simulink model "Script_es2"  (R2023b)
settings: Solver=VariableStepAuto  StartTime=0.0  StopTime=30  RelTol=1e-3
libraries: dspfdesign x8, vrlib x6
settings Model: PacingRate=4  Creator=bolla  LastModifiedBy=bolla

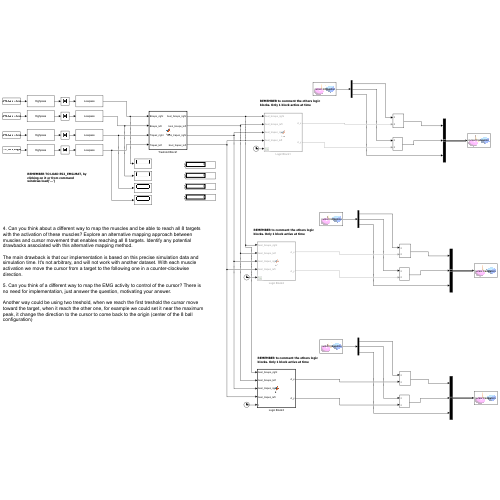
[thumbnail: Simulink's stored preview of the top-level diagram]
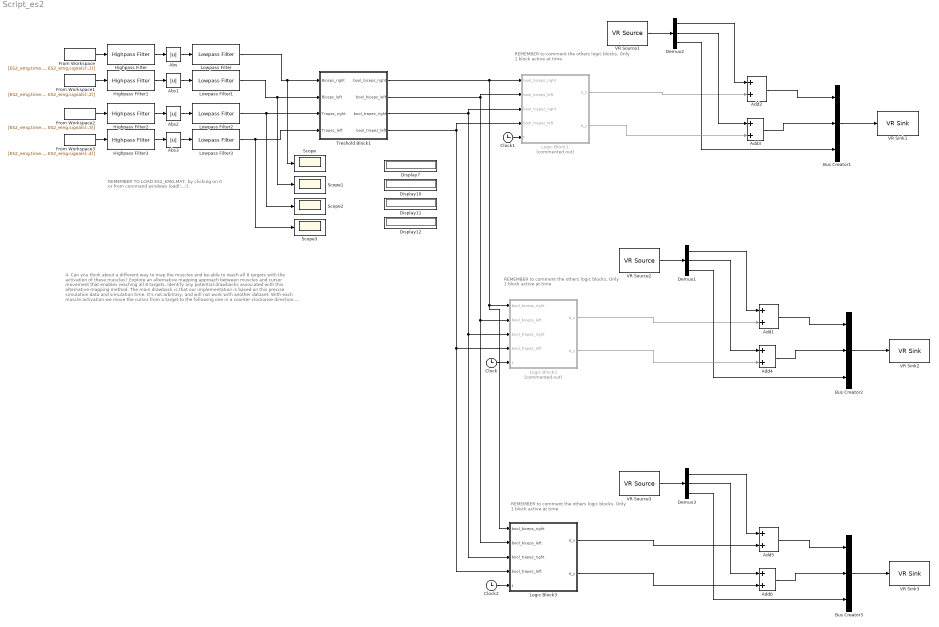
== system Script_es2 ==
  note: REMEMBER TO LOAD ES2_EMG.MAT, by clicking on it or from command windows load('...')
  note: REMEMBER to comment the others logic blocks. Only 1 block active at time
  note: 4. Can you think about a different way to map the muscles and be able to reach all 8 targets with the activation of these muscles? Explore an alternative mapping approach between muscles and cursor movement that enables reaching all 8 targets. Identify any potential drawbacks associated with this alternative mapping method.
      |
      | The main drawback is that our implementation is based on this precise simulation data and simulation time. It's not arbitrary, and will not work with another dataset. With each muscle activation we move the cursor from a target to the following one in a counter-clockwise direction.
      |
      | 5. Can you think of a different way to map the EMG activity to control of the cursor? There is no need for implementation, just answer the question, motivating your answer.
      |
      | Another way could be using two treshold, when we reach the first treshold the cursor move toward the target, when it reach the other one, for example we could set it near the maximum peak, it change the direction to the cursor to come back to the origin (center of the 8 ball configuration)
  note: REMEMBER to comment the others logic blocks. Only 1 block active at time
  note: REMEMBER to comment the others logic blocks. Only 1 block active at time
  Abs{,1..3} (4 alike) : Abs  SaturateOnIntegerOverflow=off
  Add{1..6} (6 alike) : Sum
  Bus Creator1 : BusCreator  Inputs=3
  Bus Creator2 : BusCreator  Inputs=3
  Bus Creator3 : BusCreator  Inputs=3
  Clock : Clock
  Clock1 : Clock
  Clock2 : Clock
  Demux1 : Demux  Outputs=3
  Demux2 : Demux  Outputs=3
  Demux3 : Demux  Outputs=3
  Display{7,10..12} (4 alike) : Display
  From Workspace : FromWorkspace  VariableName=[ES2_emg.time, ES2_emg.signals(:,1)]  SampleTime=0.001
  From Workspace1 : FromWorkspace  VariableName=[ES2_emg.time, ES2_emg.signals(:,2)]  SampleTime=0.001
  From Workspace2 : FromWorkspace  VariableName=[ES2_emg.time, ES2_emg.signals(:,3)]  SampleTime=0.001
  From Workspace3 : FromWorkspace  VariableName=[ES2_emg.time, ES2_emg.signals(:,4)]  SampleTime=0.001
  Highpass Filter{,1..3} (4 alike) : dspfdesign/Highpass Filter  FilterType=FIR  DesignForMinimumOrder=on  FilterOrder=50  StopbandFrequency=30  PassbandFrequency=450  StopbandAttenuation=80  PassbandRipple=0.1  SampleRate=44100  SimulateUsing=Interpreted execution  roundingMode=Floor  coeffsDataTypeStr=fixdt(1,16)
  Logic Block1 : MATLAB Function  Commented=on  TreatAsAtomicUnit=on  SystemSampleTime=0.1
  Logic Block2 : MATLAB Function  Commented=on  TreatAsAtomicUnit=on  SystemSampleTime=0.1
  Logic Block3 : MATLAB Function  TreatAsAtomicUnit=on  SystemSampleTime=0.1
  Lowpass Filter{,1..3} (4 alike) : dspfdesign/Lowpass Filter  FilterType=FIR  DesignForMinimumOrder=on  FilterOrder=50  PassbandFrequency=3  StopbandFrequency=6  PassbandRipple=0.1  StopbandAttenuation=80  SampleRate=44100  SimulateUsing=Interpreted execution  roundingMode=Floor  coeffsDataTypeStr=fixdt(1,16)
  Scope{,1..3} (4 alike) : Scope
  Treshold Block1 : MATLAB Function  TreatAsAtomicUnit=on  SystemSampleTime=0.1
  VR Sink1 : vrlib/VR Sink  InstantiateOnLoad=on  SampleTime=0.1  ViewEnable=on  RemoteChange=off  RemoteView=off  FieldsWritten=cursor.translation.3.1.1.double  WorldFileName=8_palline_color.wrl  AutoView=off  VideoDimensions=[]  AllowVariableSize=off
  VR Sink2 : vrlib/VR Sink  InstantiateOnLoad=on  SampleTime=0.1  ViewEnable=on  RemoteChange=off  RemoteView=off  FieldsWritten=cursor.translation.3.1.1.double  WorldFileName=8_palline_color.wrl  AutoView=off  VideoDimensions=[]  AllowVariableSize=off  FigureProperties="{'Position', 'Name', 'Viewpoint', 'CameraBound', 'CameraDirection', 'CameraPosition', 'CameraUpVector', 'ZoomFactor', 'Antialiasing', 'Headlight', 'Lighting', 'NavPanel', 'Sound', 'StatusBar', 'Stereo3D', 'Stereo3DCameraOffset', 'Stereo3DHIT', 'ToolBar', 'Textures', 'Transparency', 'Triad', 'Wireframe', 'NavZones', 'NavMode', 'NavSpeed', 'CaptureFileFormat', 'CaptureFileName', 'Record2DCompressMethod', 'Record2DCompressQuality', 'Record2D', 'Record2DFileName', 'Record2DFPS'; [7.7000000000000000e+02   7.5500000000000000e+01   5.1000000000000000e+02   6.2450000000000000e+02], '', '_untitled_1', 'on', [0.0000000000000000e+00   0.0000000000000000e+00  -1.0000000000000000e+00], [0.0000000000000000e+00   0.0000000000000000e+00   1.6100000000000000e+02], [0.0000000000000000e+00   1.0000000000000000e+00   0.0000000000000000e+00], [3.0912680532870748e+01], 'on', 'on', 'on', 'halfbar', 'on', 'on', 'off', [1.0000000149011612e-01], [0.0000000000000000e+00], 'on', 'on', 'on', 'none', 'off', 'off', 'fly', 'normal', 'tif', '%f_anim_%n.tif', 'auto', [7.5000000000000000e+01], 'off', '%f_anim_%n.avi', 'auto'}"
  VR Sink3 : vrlib/VR Sink  InstantiateOnLoad=on  SampleTime=0.1  ViewEnable=on  RemoteChange=off  RemoteView=off  FieldsWritten=cursor.translation.3.1.1.double  WorldFileName=8_palline_color.wrl  AutoView=off  VideoDimensions=[]  AllowVariableSize=off
  VR Source1 : vrlib/VR Source  InstantiateOnLoad=on  SampleTime=0.1  ViewEnable=on  RemoteChange=off  RemoteView=off  FieldsRead=cursor.translation.1.3.1.double  WorldFileName=8_palline_color.wrl  AutoView=off  VideoDimensions=[]  AllowVariableSize=off
  VR Source2 : vrlib/VR Source  InstantiateOnLoad=on  SampleTime=0.1  ViewEnable=on  RemoteChange=off  RemoteView=off  FieldsRead=cursor.translation.1.3.1.double  WorldFileName=8_palline_color.wrl  AutoView=off  VideoDimensions=[]  AllowVariableSize=off
  VR Source3 : vrlib/VR Source  InstantiateOnLoad=on  SampleTime=0.1  ViewEnable=on  RemoteChange=off  RemoteView=off  FieldsRead=cursor.translation.1.3.1.double  WorldFileName=8_palline_color.wrl  AutoView=off  VideoDimensions=[]  AllowVariableSize=off
  wires:
  Logic Block1/1(d_x) -> Add2/2
  Demux2/3 -> Bus Creator1/3
  Treshold Block1/2(bool_biceps_left) -> Logic Block3/2(bool_biceps_left), Logic Block2/2(bool_biceps_left), Logic Block1/2(bool_biceps_left)
  Treshold Block1/4(bool_trapez_left) -> Logic Block3/4(bool_trapez_left), Logic Block2/4(bool_trapez_left), Logic Block1/4(bool_trapez_left)
  Treshold Block1/3(bool_trapez_right) -> Logic Block3/3(bool_trapez_right), Logic Block2/3(bool_trapez_right), Logic Block1/3(bool_trapez_right)
  Add3/1 -> Bus Creator1/2
  Demux2/1 -> Add2/1
  Add2/1 -> Bus Creator1/1
  Demux2/2 -> Add3/1
  VR Source1/1 -> Demux2/1
  Bus Creator1/1 -> VR Sink1/1
  Logic Block1/2(d_y) -> Add3/2
  From Workspace/1 -> Highpass Filter/1
  Highpass Filter/1 -> Abs/1
  Abs/1 -> Lowpass Filter/1
  Lowpass Filter/1 -> Scope/1, Treshold Block1/1(Biceps_right)
  Highpass Filter1/1 -> Abs1/1
  Abs1/1 -> Lowpass Filter1/1
  From Workspace1/1 -> Highpass Filter1/1
  From Workspace3/1 -> Highpass Filter3/1
  Abs3/1 -> Lowpass Filter3/1
  Highpass Filter3/1 -> Abs3/1
  Highpass Filter2/1 -> Abs2/1
  Abs2/1 -> Lowpass Filter2/1
  From Workspace2/1 -> Highpass Filter2/1
  Lowpass Filter1/1 -> Scope1/1, Treshold Block1/2(Biceps_left)
  Lowpass Filter2/1 -> Scope2/1, Treshold Block1/3(Trapez_right)
  Lowpass Filter3/1 -> Scope3/1, Treshold Block1/4(Trapez_left)
  Demux1/1 -> Add1/1
  Bus Creator2/1 -> VR Sink2/1
  Logic Block2/1(d_x) -> Add1/2
  Demux1/2 -> Add4/1
  Add1/1 -> Bus Creator2/1
  Demux1/3 -> Bus Creator2/3
  Logic Block2/2(d_y) -> Add4/2
  Add4/1 -> Bus Creator2/2
  VR Source2/1 -> Demux1/1
  Clock/1 -> Logic Block2/5(t)
  Clock1/1 -> Logic Block1/5(t)
  Demux3/2 -> Add6/1
  Logic Block3/1(d_x) -> Add5/2
  Bus Creator3/1 -> VR Sink3/1
  Demux3/1 -> Add5/1
  Add6/1 -> Bus Creator3/2
  VR Source3/1 -> Demux3/1
  Logic Block3/2(d_y) -> Add6/2
  Demux3/3 -> Bus Creator3/3
  Add5/1 -> Bus Creator3/1
  Clock2/1 -> Logic Block3/5(t)
  Treshold Block1/1(bool_biceps_right) -> Logic Block3/1(bool_biceps_right), Logic Block2/1(bool_biceps_right), Logic Block1/1(bool_biceps_right)

== matlab function Script_es2/Logic Block2 ==
  data: d_x output; d_y output; bool_biceps_right input; bool_biceps_left input; bool_trapez_right input; bool_trapez_left input; t input

function [d_x, d_y] = fcn(bool_biceps_right,bool_biceps_left, bool_trapez_right, bool_trapez_left, t)

d_x = 0;
d_y = 0;

if t<15

    if (bool_biceps_right == 1)
    
        d_x = 0.0035;
        d_y = - 0.0035;
    end
    
    if (bool_biceps_left == 1)
    
        d_x = -0.002;
        d_y = 0.002;
    end
    
    if (bool_trapez_right == 1)
        
        d_x = 0.0145;
        d_y = 0.0145;
    end
    
    if (bool_trapez_left == 1)
        
        d_x = - 0.015;
        d_y = - 0.015;
    end
end

if t>15

    if (bool_biceps_right == 1)
    
        d_x = -0.005;
        d_y =  0.005;
    end
    
    if (bool_biceps_left == 1)
    
        d_x = 0.0025;
        d_y = - 0.0025;
    end
    
    if (bool_trapez_right == 1)
        
        d_x = -0.012;
        d_y = -0.012;
    end
    
    if (bool_trapez_left == 1)
        
        d_x =  5*0.016;
        d_y = 5* 0.015;
    end
end

== matlab function Script_es2/Logic Block3 ==
  data: d_x output; d_y output; bool_biceps_right input; bool_biceps_left input; bool_trapez_right input; bool_trapez_left input; t input

function [d_x, d_y] = fcn(bool_biceps_right,bool_biceps_left, bool_trapez_right, bool_trapez_left, t)

d_x = 0;
d_y = 0;


if t<4

    
    if (bool_trapez_right == 1)
    
        d_x = 0.02;
    end
    
    
end


if t>4 && t<15

     if (bool_trapez_left == 1)
        
        d_x = - 0.006;
        d_y = 0.015;
     end

    if (bool_biceps_right == 1)
    
        d_x = -0.0035;
        d_y =  0.0015;
    end
    
    if (bool_biceps_left == 1)
    
        d_x = -0.002;
        d_y = -0.001;
    end
    
    
end

if t>15

     if (bool_trapez_right == 1)
        
        d_x = -0.005;
        d_y = - 0.012;
     end

    if (bool_trapez_left == 1)
        
        d_x =  0.041;
        d_y = - 0.063;
    end

    

    if (bool_biceps_right == 1)
    
        d_x = 0.0038;
        d_y =  -0.0028;
    end
    
    if (bool_biceps_left == 1)
    
        d_x = 0.0025;
        d_y =  0.0015;
    end
        
end

== matlab function Script_es2/Treshold Block1 ==
  data: bool_biceps_right output; Biceps_right input; Biceps_left input; Trapez_right input; Trapez_left input; bool_biceps_left output; bool_trapez_right output; bool_trapez_left output

function [bool_biceps_right,bool_biceps_left, bool_trapez_right, bool_trapez_left] = fcn(Biceps_right,Biceps_left, Trapez_right, Trapez_left)


bool_biceps_right = 0;
bool_biceps_left = 0;
bool_trapez_right = 0;
bool_trapez_left = 0;
 

    if Biceps_right > 0.0065      % settare bene i treshold per la sensibilità
        bool_biceps_right = 1;
        % biceps_left = 0;
        % trapez_right = 0;
        % trapez_left = 0;

    elseif Biceps_left > 0.003
        % biceps_right = 0 ;
       bool_biceps_left = 1;
        % trapez_right = 0;
        % trapez_left = 0;

    elseif Trapez_right > 0.01
        % biceps_right = 0 ;
        % biceps_left = 0;
        bool_trapez_right = 1;
        % trapez_left = 0;

    elseif Trapez_left > 0.0075
        %  biceps_right = 0 ;
        % biceps_left = 0;
        % trapez_right = 0;
        bool_trapez_left = 1;
    % else
    %     bool_biceps_right = 0;
    %     bool_biceps_left = 0;
    %     bool_trapez_right = 0;
    %     bool_trapez_left = 0;

  
    end


%figure(2)
%subplot(4,1,1)
%plot(biceps_right)
%subplot(4,1,2)
%plot(biceps_left)
%subplot(4,1,3)
%plot(trapez_right)
%subplot(4,1,4)
%plot(trapez_left)

== matlab function Script_es2/Logic Block1 ==
  data: d_x output; d_y output; bool_biceps_right input; bool_biceps_left input; bool_trapez_right input; bool_trapez_left input; t input

function [d_x, d_y] = fcn(bool_biceps_right,bool_biceps_left, bool_trapez_right, bool_trapez_left,t)

d_x = 0;
d_y = 0;

if t<15

    if (bool_biceps_right == 1)
    
        d_x = 0.005;
    end
    
    if (bool_biceps_left == 1)
    
        d_x = -0.0056/2;
    end
    
    if (bool_trapez_right == 1)
    
        d_y = 0.02;
    end
    
    if (bool_trapez_left == 1)
    
        d_y = -0.02;
    end
end

if t>15

    if (bool_biceps_right == 1)
    
        d_x = -0.0065;
    end
    
    if (bool_biceps_left == 1)
    
        d_x = +0.003;
    end
    
    if (bool_trapez_right == 1)
    
        d_y = -0.016;
    end
    
    if (bool_trapez_left == 1)
    
        d_y = 0.095;
    end
end
